simulink model "SIRComp"  (R2020a)
settings: Solver=ode45  StartTime=0.0  StopTime=5  MaxStep=0.01  RelTol=1e-3
values from neighbouring files (symbols this model uses):
  beta = X(1)    [ErroQuadratico.m]    (also in ErroQuadraticoSIR.m)
  I0 = 2    [ErroQuadratico.m]    (also in ErroQuadraticoSIR.m)
  r = X(2)    [ErroQuadratico.m]    (also in ErroQuadraticoSIR.m)
  R0 = 0    [ErroQuadratico.m]    (also in ErroQuadraticoSIR.m)
  S0 = 60e6    (= 60000000)    [ErroQuadratico.m]    (also in ErroQuadraticoSIR.m)
undefined symbols (not defined in the file or in its folder): A, B, C, D, x0
settings Model: Creator=a1  LastModifiedBy=a1
settings SolverCC: InitialStep=0.01

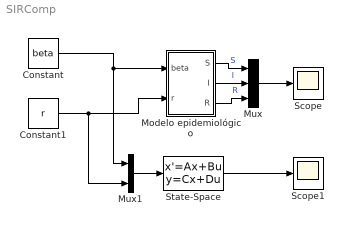
== system SIRComp ==
  Constant : Constant  Value=beta
  Constant1 : Constant  Value=r
  Modelo epidemiológico : Subsystem
  Mux : Mux  Inputs=3
  Mux1 : Mux  Inputs=2
  Scope : Scope
  Scope1 : Scope
  State-Space : StateSpace  A=A  B=B  C=C  D=D  InitialCondition=x0
  wires:
  Constant/1 -> Mux1/1, Modelo epidemiológico/1(beta)
  Constant1/1 -> Mux1/2, Modelo epidemiológico/2(r)
  Modelo epidemiológico/2(I) -> Mux/2  "I"
  Modelo epidemiológico/1(S) -> Mux/1  "S"
  Modelo epidemiológico/3(R) -> Mux/3  "R"
  Mux/1 -> Scope/1
  Mux1/1 -> State-Space/1
  State-Space/1 -> Scope1/1

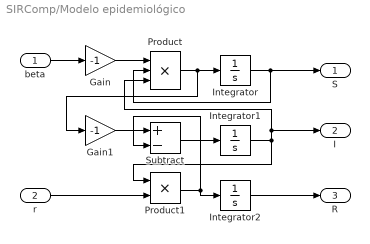
== system SIRComp/Modelo epidemiológico ==
  beta : Inport
  r : Inport  Port=2
  Gain : Gain  Gain=-1
  Gain1 : Gain  Gain=-1
  Integrator : Integrator  InitialCondition=S0
  Integrator1 : Integrator  InitialCondition=I0
  Integrator2 : Integrator  InitialCondition=R0
  Product : Product  Inputs=3
  Product1 : Product
  Subtract : Sum  Inputs=+-
  S : Outport
  I : Outport  Port=2
  R : Outport  Port=3
  wires:
  beta/1 -> Gain/1
  Gain1/1 -> Subtract/1
  Integrator2/1 -> R/1
  Gain/1 -> Product/1
  Product1/1 -> Integrator2/1, Subtract/2
  Subtract/1 -> Integrator1/1
  Product/1 -> Gain1/1, Integrator/1
  r/1 -> Product1/2
  Integrator/1 -> S/1, Product/2
  Integrator1/1 -> Product1/1, I/1, Product/3
